simulink model "ControllerDesignNonLinear"  (R2019b)
settings: Solver=VariableStepAuto  StartTime=0.0  StopTime=25  RelTol=1e-3
libraries: simulink x3
settings Model: Creator=Bekircan Keceoglu  LastModifiedBy=Bekircan Keceoglu

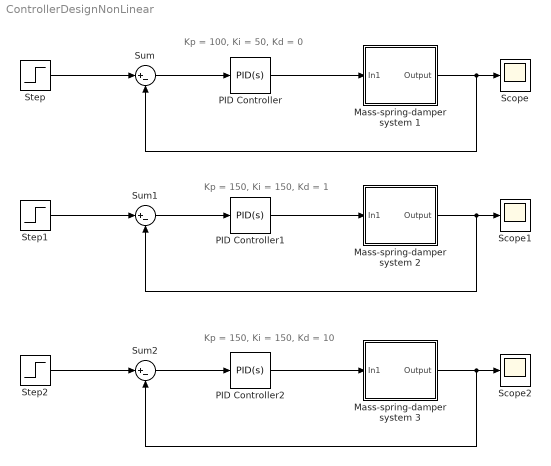
== system ControllerDesignNonLinear ==
  note: Kp = 100, Ki = 50, Kd = 0
  note: Kp = 150, Ki = 150, Kd = 1
  note: Kp = 150, Ki = 150, Kd = 10
  Mass-spring-damper system 1 : Subsystem
  Mass-spring-damper system 2 : Subsystem
  Mass-spring-damper system 3 : Subsystem
  PID Controller : simulink/Continuous/PID Controller  Controller=PID  Form=Parallel  TimeDomain=Continuous-time  SampleTime=-1  IntegratorMethod=Forward Euler  FilterMethod=Forward Euler  ControllerParametersSource=internal  P=100  I=50  D=0  UseFilter=on  N=100  TunerSelectOption=Transfer Function Based (PID Tuner App)  InitialConditionSource=internal  InitialConditionForIntegrator=0  InitialConditionForFilter=0  DifferentiatorICPrevScaledInput=0  ExternalReset=none  TrackingMode=off  Kt=1  LimitOutput=off  UpperSaturationLimit=inf  LowerSaturationLimit=-inf  LinearizeAsGain=on  AntiWindupMode=none  Kb=1  POutMin=[]  POutMax=[]  IOutMin=[]  IOutMax=[]  DOutMin=[]  DOutMax=[]  NOutMin=[]  NOutMax=[]  SumOutMin=[]  SumOutMax=[]  SaturationOutMin=[]  SaturationOutMax=[]  PParamMin=[]  PParamMax=[]  IParamMin=[]  IParamMax=[]  DParamMin=[]  DParamMax=[]  NParamMin=[]  NParamMax=[]  KbParamMin=[]  KbParamMax=[]  KtParamMin=[]  KtParamMax=[]  KbOutMin=[]  KbOutMax=[]  KtOutMin=[]  KtOutMax=[]  IntegratorOutMin=[]  IntegratorOutMax=[]  FilterOutMin=[]  FilterOutMax=[]  SumI1OutMin=[]  SumI1OutMax=[]  SumI2OutMin=[]  SumI2OutMax=[]  SumI3OutMin=[]  SumI3OutMax=[]  SumI4OutMin=[]  SumI4OutMax=[]  SumDOutMin=[]  SumDOutMax=[]  DifferentiatorOutMin=[]  DifferentiatorOutMax=[]  FilterDiffOutCoefMin=[]  FilterDiffOutCoefMax=[]  ReciprocalOutMin=[]  ReciprocalOutMax=[]  SumDenOutMin=[]  SumDenOutMax=[]  SumNumOutMin=[]  SumNumOutMax=[]  DivideOutMin=[]  DivideOutMax=[]  IntegratorContinuousStateAttributes=''  IntegratorStateMustResolveToSignalObject=off  IntegratorRTWStateStorageClass=Auto  FilterContinuousStateAttributes=''  FilterStateMustResolveToSignalObject=off  FilterRTWStateStorageClass=Auto  ParallelPVariant=InternalParameters  IdealPVariant=Disabled  IVariant=InternalParameters  DVariant=InternalParameters  IntegratorVariant=Continuous  SatVariant=Disabled  AWVariant=Passthrough  PCopyVariant=Disabled  TRVariant=Disabled  FdbkBlocksVariant=Forward  IdealPFdbkVariant=Disabled  SatFdbkVariant=Disabled  DerivativeFilterVariant=ContFilter  NVariant=InternalParameters  NCopyVariant=Disabled  FilterICVariant=InternalICsFilter  IntegratorICVariant=InternalICs  ExternalResetVariant=Disabled  TRSumVariant=Passthrough  SumFdbkVariant=Disabled  SumVariant=Sum_PID
  PID Controller1 : simulink/Continuous/PID Controller  Controller=PID  Form=Parallel  TimeDomain=Continuous-time  SampleTime=-1  IntegratorMethod=Forward Euler  FilterMethod=Forward Euler  ControllerParametersSource=internal  P=150  I=150  D=1  UseFilter=on  N=100  TunerSelectOption=Transfer Function Based (PID Tuner App)  InitialConditionSource=internal  InitialConditionForIntegrator=0  InitialConditionForFilter=0  DifferentiatorICPrevScaledInput=0  ExternalReset=none  TrackingMode=off  Kt=1  LimitOutput=off  UpperSaturationLimit=inf  LowerSaturationLimit=-inf  LinearizeAsGain=on  AntiWindupMode=none  Kb=1  POutMin=[]  POutMax=[]  IOutMin=[]  IOutMax=[]  DOutMin=[]  DOutMax=[]  NOutMin=[]  NOutMax=[]  SumOutMin=[]  SumOutMax=[]  SaturationOutMin=[]  SaturationOutMax=[]  PParamMin=[]  PParamMax=[]  IParamMin=[]  IParamMax=[]  DParamMin=[]  DParamMax=[]  NParamMin=[]  NParamMax=[]  KbParamMin=[]  KbParamMax=[]  KtParamMin=[]  KtParamMax=[]  KbOutMin=[]  KbOutMax=[]  KtOutMin=[]  KtOutMax=[]  IntegratorOutMin=[]  IntegratorOutMax=[]  FilterOutMin=[]  FilterOutMax=[]  SumI1OutMin=[]  SumI1OutMax=[]  SumI2OutMin=[]  SumI2OutMax=[]  SumI3OutMin=[]  SumI3OutMax=[]  SumI4OutMin=[]  SumI4OutMax=[]  SumDOutMin=[]  SumDOutMax=[]  DifferentiatorOutMin=[]  DifferentiatorOutMax=[]  FilterDiffOutCoefMin=[]  FilterDiffOutCoefMax=[]  ReciprocalOutMin=[]  ReciprocalOutMax=[]  SumDenOutMin=[]  SumDenOutMax=[]  SumNumOutMin=[]  SumNumOutMax=[]  DivideOutMin=[]  DivideOutMax=[]  IntegratorContinuousStateAttributes=''  IntegratorStateMustResolveToSignalObject=off  IntegratorRTWStateStorageClass=Auto  FilterContinuousStateAttributes=''  FilterStateMustResolveToSignalObject=off  FilterRTWStateStorageClass=Auto  ParallelPVariant=InternalParameters  IdealPVariant=Disabled  IVariant=InternalParameters  DVariant=InternalParameters  IntegratorVariant=Continuous  SatVariant=Disabled  AWVariant=Passthrough  PCopyVariant=Disabled  TRVariant=Disabled  FdbkBlocksVariant=Forward  IdealPFdbkVariant=Disabled  SatFdbkVariant=Disabled  DerivativeFilterVariant=ContFilter  NVariant=InternalParameters  NCopyVariant=Disabled  FilterICVariant=InternalICsFilter  IntegratorICVariant=InternalICs  ExternalResetVariant=Disabled  TRSumVariant=Passthrough  SumFdbkVariant=Disabled  SumVariant=Sum_PID
  PID Controller2 : simulink/Continuous/PID Controller  Controller=PID  Form=Parallel  TimeDomain=Continuous-time  SampleTime=-1  IntegratorMethod=Forward Euler  FilterMethod=Forward Euler  ControllerParametersSource=internal  P=150  I=150  D=10  UseFilter=on  N=100  TunerSelectOption=Transfer Function Based (PID Tuner App)  InitialConditionSource=internal  InitialConditionForIntegrator=0  InitialConditionForFilter=0  DifferentiatorICPrevScaledInput=0  ExternalReset=none  TrackingMode=off  Kt=1  LimitOutput=off  UpperSaturationLimit=inf  LowerSaturationLimit=-inf  LinearizeAsGain=on  AntiWindupMode=none  Kb=1  POutMin=[]  POutMax=[]  IOutMin=[]  IOutMax=[]  DOutMin=[]  DOutMax=[]  NOutMin=[]  NOutMax=[]  SumOutMin=[]  SumOutMax=[]  SaturationOutMin=[]  SaturationOutMax=[]  PParamMin=[]  PParamMax=[]  IParamMin=[]  IParamMax=[]  DParamMin=[]  DParamMax=[]  NParamMin=[]  NParamMax=[]  KbParamMin=[]  KbParamMax=[]  KtParamMin=[]  KtParamMax=[]  KbOutMin=[]  KbOutMax=[]  KtOutMin=[]  KtOutMax=[]  IntegratorOutMin=[]  IntegratorOutMax=[]  FilterOutMin=[]  FilterOutMax=[]  SumI1OutMin=[]  SumI1OutMax=[]  SumI2OutMin=[]  SumI2OutMax=[]  SumI3OutMin=[]  SumI3OutMax=[]  SumI4OutMin=[]  SumI4OutMax=[]  SumDOutMin=[]  SumDOutMax=[]  DifferentiatorOutMin=[]  DifferentiatorOutMax=[]  FilterDiffOutCoefMin=[]  FilterDiffOutCoefMax=[]  ReciprocalOutMin=[]  ReciprocalOutMax=[]  SumDenOutMin=[]  SumDenOutMax=[]  SumNumOutMin=[]  SumNumOutMax=[]  DivideOutMin=[]  DivideOutMax=[]  IntegratorContinuousStateAttributes=''  IntegratorStateMustResolveToSignalObject=off  IntegratorRTWStateStorageClass=Auto  FilterContinuousStateAttributes=''  FilterStateMustResolveToSignalObject=off  FilterRTWStateStorageClass=Auto  ParallelPVariant=InternalParameters  IdealPVariant=Disabled  IVariant=InternalParameters  DVariant=InternalParameters  IntegratorVariant=Continuous  SatVariant=Disabled  AWVariant=Passthrough  PCopyVariant=Disabled  TRVariant=Disabled  FdbkBlocksVariant=Forward  IdealPFdbkVariant=Disabled  SatFdbkVariant=Disabled  DerivativeFilterVariant=ContFilter  NVariant=InternalParameters  NCopyVariant=Disabled  FilterICVariant=InternalICsFilter  IntegratorICVariant=InternalICs  ExternalResetVariant=Disabled  TRSumVariant=Passthrough  SumFdbkVariant=Disabled  SumVariant=Sum_PID
  Scope : Scope
  Scope1 : Scope
  Scope2 : Scope
  Step : Step  SampleTime=0
  Step1 : Step  SampleTime=0
  Step2 : Step  SampleTime=0
  Sum : Sum  Inputs=|+-
  Sum1 : Sum  Inputs=|+-
  Sum2 : Sum  Inputs=|+-
  wires:
  PID Controller/1 -> Mass-spring-damper system 1/1(In1)
  Sum/1 -> PID Controller/1
  Mass-spring-damper system 1/1(Output) -> Sum/2, Scope/1
  Step/1 -> Sum/1
  Step1/1 -> Sum1/1
  PID Controller1/1 -> Mass-spring-damper system 2/1(In1)
  Mass-spring-damper system 2/1(Output) -> Sum1/2, Scope1/1
  Sum1/1 -> PID Controller1/1
  Mass-spring-damper system 3/1(Output) -> Sum2/2, Scope2/1
  Step2/1 -> Sum2/1
  PID Controller2/1 -> Mass-spring-damper system 3/1(In1)
  Sum2/1 -> PID Controller2/1

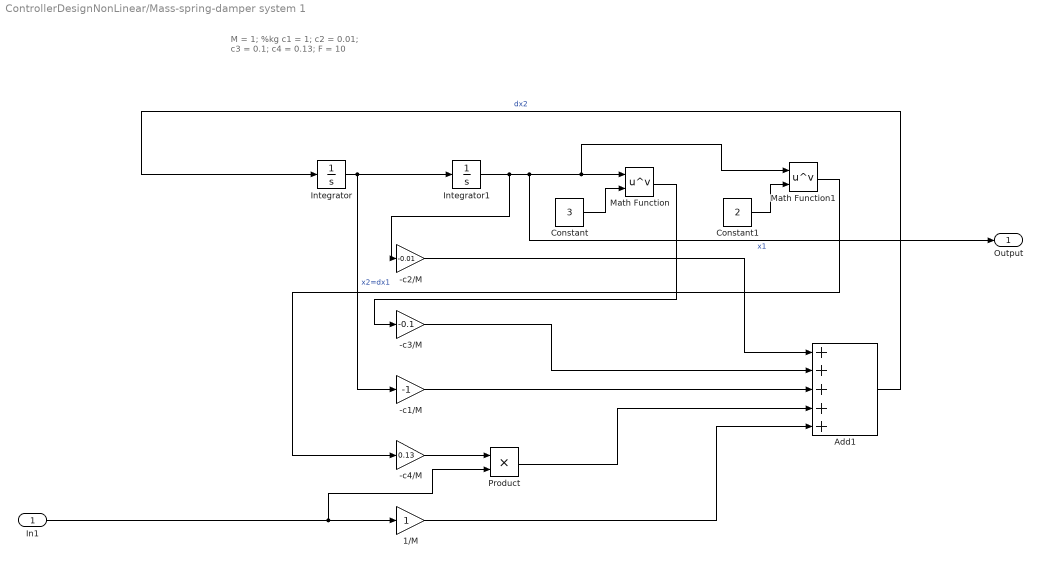
== system ControllerDesignNonLinear/Mass-spring-damper system 1 ==
  note: M  = 1; %kg
      | c1 = 1;
      | c2 = 0.01;
      | c3 = 0.1;
      | c4 = 0.13;
      | F  = 10
  In1 : Inport
  -c1/M : Gain  Gain=-1
  -c2/M : Gain  Gain=-0.01
  -c3/M : Gain  Gain=-0.1
  -c4/M : Gain  Gain=0.13
  1/M : Gain
  Add1 : Sum  Inputs=+++++
  Constant : Constant  Value=3
  Constant1 : Constant  Value=2
  Integrator : Integrator  InitialCondition=5
  Integrator1 : Integrator
  Math Function : Math  Operator=pow  SignedPower=off  SaturateOnIntegerOverflow=on
  Math Function1 : Math  Operator=pow  SignedPower=off  SaturateOnIntegerOverflow=on
  Product : Product
  Output : Outport
  wires:
  Integrator1/1 -> -c2/M/1, Output/1, Math Function1/1, Math Function/1  "x1"
  Math Function/1 -> -c3/M/1
  Constant/1 -> Math Function/2
  -c3/M/1 -> Add1/2
  Product/1 -> Add1/4
  -c1/M/1 -> Add1/3
  -c4/M/1 -> Product/1
  Math Function1/1 -> -c4/M/1
  Constant1/1 -> Math Function1/2
  -c2/M/1 -> Add1/1
  In1/1 -> Product/2, 1/M/1
  Integrator/1 -> -c1/M/1, Integrator1/1  "x2=dx1"
  Add1/1 -> Integrator/1  "dx2"
  1/M/1 -> Add1/5

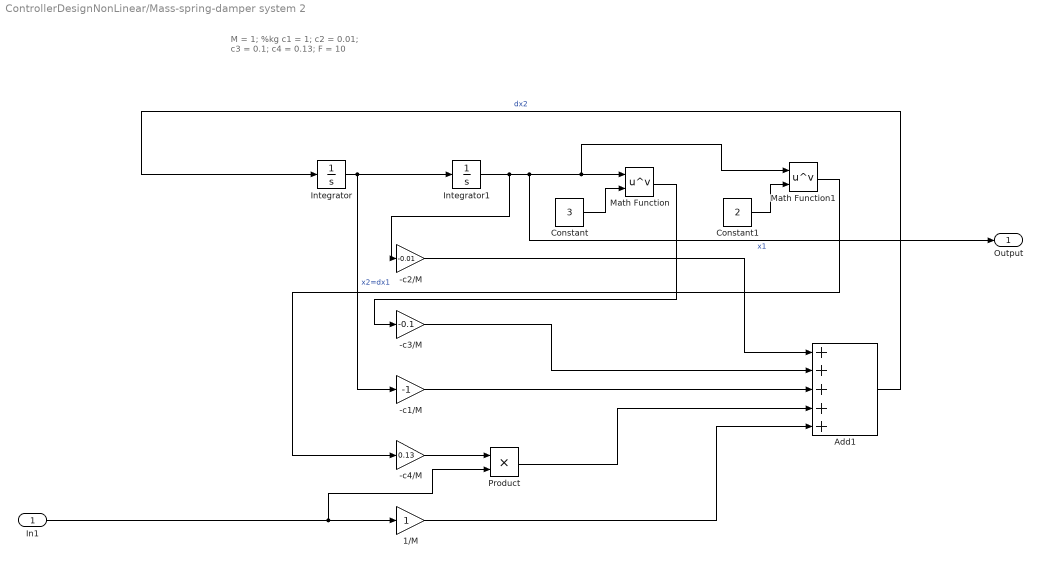
== system ControllerDesignNonLinear/Mass-spring-damper system 2 ==
  note: M  = 1; %kg
      | c1 = 1;
      | c2 = 0.01;
      | c3 = 0.1;
      | c4 = 0.13;
      | F  = 10
  In1 : Inport
  -c1/M : Gain  Gain=-1
  -c2/M : Gain  Gain=-0.01
  -c3/M : Gain  Gain=-0.1
  -c4/M : Gain  Gain=0.13
  1/M : Gain
  Add1 : Sum  Inputs=+++++
  Constant : Constant  Value=3
  Constant1 : Constant  Value=2
  Integrator : Integrator  InitialCondition=5
  Integrator1 : Integrator
  Math Function : Math  Operator=pow  SignedPower=off  SaturateOnIntegerOverflow=on
  Math Function1 : Math  Operator=pow  SignedPower=off  SaturateOnIntegerOverflow=on
  Product : Product
  Output : Outport
  wires:
  Integrator1/1 -> -c2/M/1, Output/1, Math Function1/1, Math Function/1  "x1"
  Math Function/1 -> -c3/M/1
  Constant/1 -> Math Function/2
  -c3/M/1 -> Add1/2
  Product/1 -> Add1/4
  -c1/M/1 -> Add1/3
  -c4/M/1 -> Product/1
  Math Function1/1 -> -c4/M/1
  Constant1/1 -> Math Function1/2
  -c2/M/1 -> Add1/1
  In1/1 -> Product/2, 1/M/1
  Integrator/1 -> -c1/M/1, Integrator1/1  "x2=dx1"
  Add1/1 -> Integrator/1  "dx2"
  1/M/1 -> Add1/5

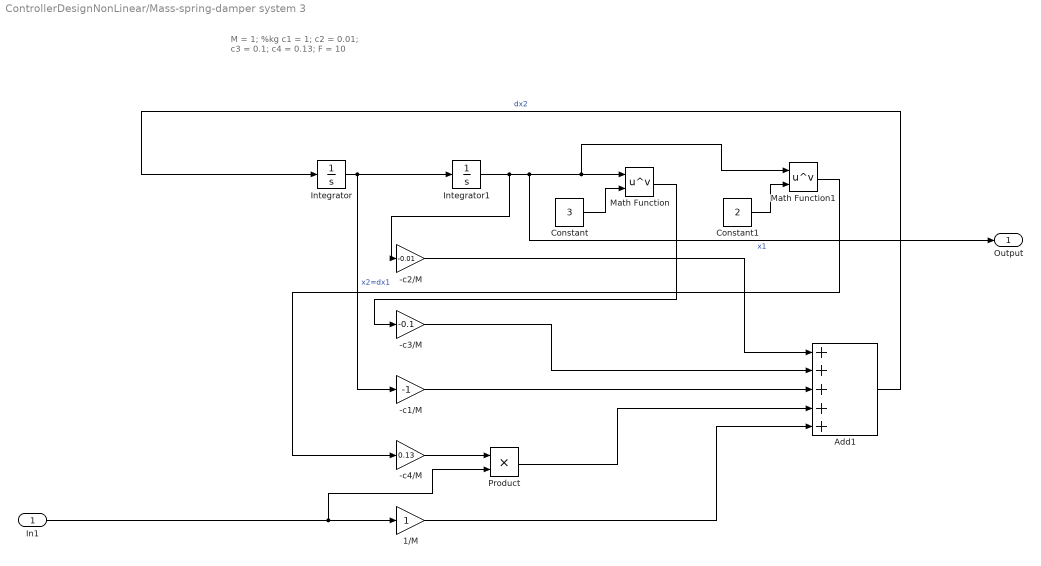
== system ControllerDesignNonLinear/Mass-spring-damper system 3 ==
  note: M  = 1; %kg
      | c1 = 1;
      | c2 = 0.01;
      | c3 = 0.1;
      | c4 = 0.13;
      | F  = 10
  In1 : Inport
  -c1/M : Gain  Gain=-1
  -c2/M : Gain  Gain=-0.01
  -c3/M : Gain  Gain=-0.1
  -c4/M : Gain  Gain=0.13
  1/M : Gain
  Add1 : Sum  Inputs=+++++
  Constant : Constant  Value=3
  Constant1 : Constant  Value=2
  Integrator : Integrator  InitialCondition=5
  Integrator1 : Integrator
  Math Function : Math  Operator=pow  SignedPower=off  SaturateOnIntegerOverflow=on
  Math Function1 : Math  Operator=pow  SignedPower=off  SaturateOnIntegerOverflow=on
  Product : Product
  Output : Outport
  wires:
  Integrator1/1 -> -c2/M/1, Output/1, Math Function1/1, Math Function/1  "x1"
  Math Function/1 -> -c3/M/1
  Constant/1 -> Math Function/2
  -c3/M/1 -> Add1/2
  Product/1 -> Add1/4
  -c1/M/1 -> Add1/3
  -c4/M/1 -> Product/1
  Math Function1/1 -> -c4/M/1
  Constant1/1 -> Math Function1/2
  -c2/M/1 -> Add1/1
  In1/1 -> Product/2, 1/M/1
  Integrator/1 -> -c1/M/1, Integrator1/1  "x2=dx1"
  Add1/1 -> Integrator/1  "dx2"
  1/M/1 -> Add1/5
